simulink model "Model_3D"  (R2020b)
settings: Solver=ode8  StartTime=0.0  StopTime=3  FixedStep=0.005  RelTol=1e-3
values from neighbouring files (symbols this model uses):
  Am = [1 8 10]    [my_config_1213.mat]    (also in my_config_1219.mat)
  Bm = [1 10]    [my_config_1213.mat]    (also in my_config_1219.mat)
  cc = [1 0.92774349 0.86070798 0.79851622 0.74081822 0.68728928 0.63762815 0.59155536 0.54881164 0.50915642 0.47236655 0.43823499 ... (41 elements, 1x41)]    [my_config_1213.mat]    (also in my_config_1219.mat)
  cc_new = [1 0.92774349 0.86070798 0.79851622 0.74081822 0.68728928 0.63762815 0.59155536 0.54881164 0.50915642 0.47236655 0.43823499 ... (41 elements, 1x41)]    [my_config_1213.mat]    (also in my_config_1219.mat)
  D = [64.807 64.807 64.807]    [my_config_1213.mat]    (also in my_config_1219.mat)
  g1 = [-1 0 1]    [my_config_1213.mat]
  g2 = [-1 0.6 1]    [my_config_1213.mat]
  gamma1 = 1.2    [my_config_1213.mat]    (also in my_config_1219.mat)
  gamma2 = 0.5    [my_config_1213.mat]    (also in my_config_1219.mat)
  K = [1050 1050 1050]    [my_config_1213.mat]    (also in my_config_1219.mat; my_config_1224.mat)
  left_0 = [0 0 0]    [my_config_1219.mat]
  m1 = 1    [my_config_1213.mat]    (also in my_config_1219.mat; my_config_1224.mat)
  m2 = 1    [my_config_1213.mat]    (also in my_config_1219.mat; my_config_1224.mat)
  right_0 = [0 0.6 0]    [my_config_1213.mat]    (also in my_config_1219.mat)
  tau1 = 3    [my_config_1213.mat]    (also in my_config_1219.mat)
  weight = [0.0266866854 0.00199886353 0 0.185908993 0.0191898792 0 0.285018336 0.0372844837 0 0.420259935 0.0646488362 0 ... (123 elements, 3x41)]    [my_config_1213.mat]    (also in my_config_1219.mat)
  width = [191.53405062 222.53081866 258.54392519 300.38518553 348.99779456 405.47758835 471.09774681 547.33749391 635.91544276 738.82833688 858.39606128 997.31393782 ... (41 elements, 1x41)]    [my_config_1213.mat]    (also in my_config_1219.mat)
  width_new = [191.53405062 222.53081866 258.54392519 300.38518553 348.99779456 405.47758835 471.09774681 547.33749391 635.91544276 738.82833688 858.39606128 997.31393782 ... (41 elements, 1x41)]    [my_config_1213.mat]    (also in my_config_1219.mat)
  x1_0 = [0 0.2 0]    [my_config_1213.mat]    (also in my_config_1219.mat; my_config_1224.mat)
  x2_0 = [0 0.4 0]    [my_config_1213.mat]    (also in my_config_1219.mat; my_config_1224.mat)
undefined symbols (not defined in the file or in its folder): b1, b2, b3, k1, k2, k3
settings Model: Creator=nathan  LastModifiedBy=10788
settings OptimizationCC: DefaultParameterBehavior=Inlined  EnhancedBackFolding=on  PassReuseOutputArgsAs=Individual arguments  ZeroExternalMemoryAtStartup=off  ZeroInternalMemoryAtStartup=off  OptimizeBlockOrder=speed  DifferentSizesBufferReuse=on  OptimizationCustomize=off  EfficientTunableParamExpr=on
settings DebuggingCC: ParameterTunabilityLossMsg=error
settings SFSimCC: MATLABDynamicMemAlloc=off  SimTargetLang=C++
settings RTWCC: Description=Create Visual C/C++ Solution File for Embedded Coder  SystemTargetFile=ert.tlc  GenCodeOnly=on  TemplateMakefile=RTW.MSVCBuild  GenerateReport=on  IncludeHyperlinkInReport=on  LaunchReport=on  TargetLang=C++  GenerateTraceInfo=on  GenerateTraceReport=on  GenerateTraceReportSl=on  GenerateTraceReportSf=on  GenerateTraceReportEml=on
settings CodeAppCC: ForceParamTrailComments=on  IgnoreCustomStorageClasses=off  OperatorAnnotations=on  SimulinkDataObjDesc=on  SFDataObjDesc=on  InsertBlockDesc=on
settings ERTTargetCC: TargetLangStandard=C++03 (ISO)  GenerateSampleERTMain=on  CodeInterfacePackaging=C++ class  SupportContinuousTime=on  InlinedParameterPlacement=NonHierarchical  RootIOFormat=Structure reference  ERTCustomFileTemplate=example_file_process.tlc

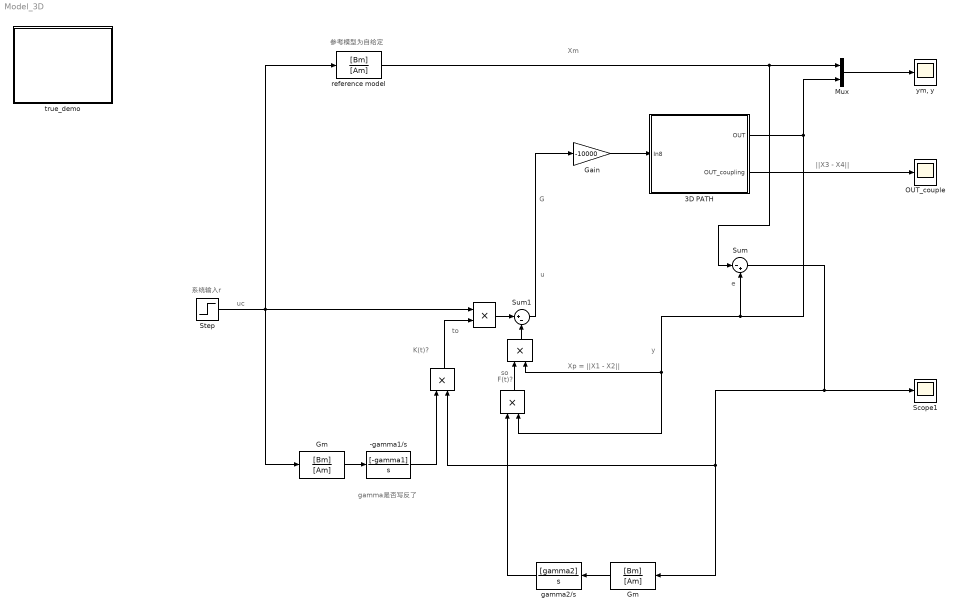
== system Model_3D ==
  note: 参考模型为自给定
  note: 系统输入r
  note: gamma是否写反了
  note: F(t)?
  note: K(t)?
  note: Xp = ||X1 - X2||
  note: ||X3 - X4||
  note: y
  note: u
  note: e
  note: so
  note: to
  note: uc
  note: Xm
  note: G
  " " : Product
  " " : Product
  "  " : Product
  "     " : Product
  -gamma1/s : TransferFcn  Numerator=[-gamma1]  Denominator=[1 0]
  3D PATH : Subsystem
  Gain : Gain  Gain=-10000
  "Gm " : TransferFcn  Numerator=[Bm]  Denominator=[Am]
  "Gm  " : TransferFcn  Numerator=[Bm]  Denominator=[Am]
  Mux : Mux  Inputs=2
  OUT_couple : Scope
  Scope1 : Scope
  Step : Step  Time=0  After=0.2  SampleTime=0
  Sum : Sum  Inputs=|-+
  Sum1 : Sum  Inputs=|+-
  gamma2/s : TransferFcn  Numerator=[gamma2]  Denominator=[1 0]
  reference model : TransferFcn  Numerator=[Bm]  Denominator=[Am]
  true_demo : Subsystem
  "ym, y" : Scope
  wires:
  3D PATH/1(OUT) -> "  "/2, " "/2, Sum/2, Mux/2
  " "/1 -> Sum1/2
  Step/1 -> "Gm  "/1, reference model/1, "     "/1
  "  "/1 -> " "/1
  Gain/1 -> 3D PATH/1(In8)
  Sum1/1 -> Gain/1
  -gamma1/s/1 -> " "/1
  " "/1 -> "     "/2
  "Gm "/1 -> gamma2/s/1
  "     "/1 -> Sum1/1
  reference model/1 -> Sum/1, Mux/1
  Mux/1 -> "ym, y"/1
  gamma2/s/1 -> "  "/1
  Sum/1 -> "Gm "/1, " "/2, Scope1/1
  "Gm  "/1 -> -gamma1/s/1
  3D PATH/2(OUT_coupling) -> OUT_couple/1

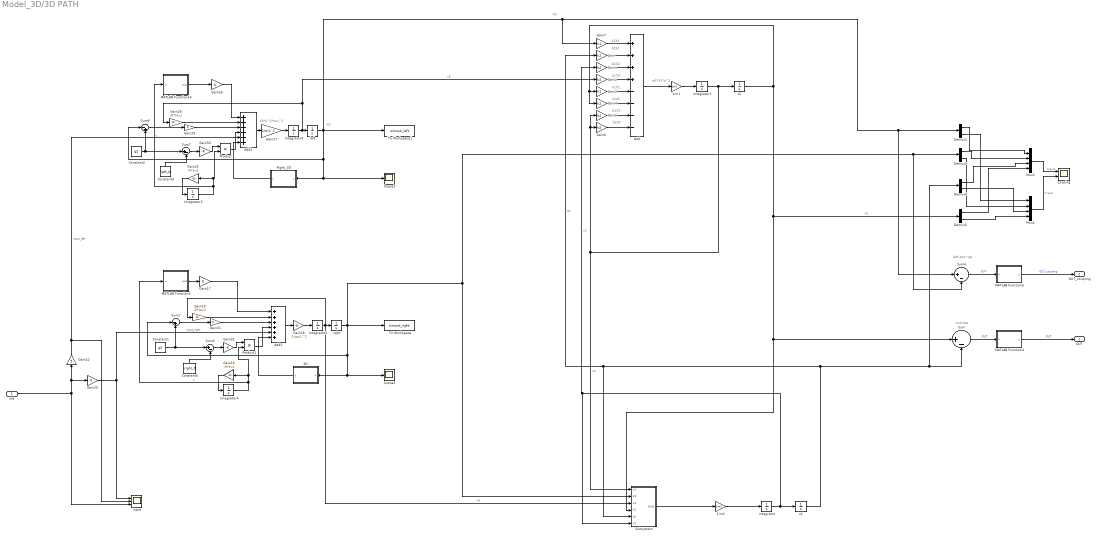
== system Model_3D/3D PATH ==
  note: X3*s^2*tau^2
  note: m1*X1*s^2
  note: k1X3
  note: X3
  note: mid two
  note: left and rigt
  note: X3
  note: k2X2
  note: b2X2'
  note: b1X3'
  note: k1X1
  note: k2X1
  note: b1X1'
  note: b2X1'
  In8 : Inport
  1/m1 : Gain  Gain=1/m1
  1/m2 : Gain  Gain=1/m2
  3D : MATLAB Function  TreatAsAtomicUnit=on
  Add : Sum  Inputs=++++----
  Add2 : Sum  Inputs=++++++
  Add4 : Sum  Inputs=++++++
  Constant1 : Constant  Value=g2
  Constant2 : Constant  Value=g1
  Constant4 : Constant  Value=left_0
  Constant5 : Constant  Value=right_0
  Demux{2..5} (4 alike) : Demux  Outputs=2
  Gain : Gain  Gain=k2
  Gain1 : Gain  Gain=b2
  Gain16 : Gain  Gain=-3/tau1
  Gain{17,26,29,31} (4 alike) : Gain  Gain=K
  Gain18 : Gain  Gain=1/tau1^2
  Gain19 : Gain  Gain=-D*tau1
  Gain2 : Gain  Gain=b1
  Gain20 : Gain  Gain=-5
  Gain22 : Gain  Gain=5
  Gain25 : Gain  Gain=-3/tau1
  Gain27 : Gain  Gain=1/tau1^2
  Gain28 : Gain  Gain=-D*tau1
  Gain3 : Gain  Gain=k1
  Gain30 : Gain  Gain=-K
  Gain32 : Gain  Gain=-K
  Gain4 : Gain  Gain=k2
  Gain5 : Gain  Gain=b1
  Gain6 : Gain  Gain=b2
  Gain7 : Gain  Gain=k1
  Integrator{,1,3,5} (4 alike) : Integrator
  Integrator2 : Integrator  InitialCondition=1
  Integrator4 : Integrator  InitialCondition=1
  MATLAB Function14 : MATLAB Function  TreatAsAtomicUnit=on
  MATLAB Function2 : MATLAB Function  TreatAsAtomicUnit=on
  MATLAB Function4 : MATLAB Function  TreatAsAtomicUnit=on
  MATLAB Function5 : MATLAB Function  TreatAsAtomicUnit=on
  Mux3 : Mux
  Mux4 : Mux
  Product : Product
  Product1 : Product
  Right_3D : MATLAB Function  TreatAsAtomicUnit=on
  Scope3 : Scope
  Scope4 : Scope
  Subsystem : Subsystem
  Sum{,3..4,7} (4 alike) : Sum  Inputs=|+-
  Sum2 : Sum  Inputs=|-+
  Sum6 : Sum  Inputs=|-+
  To Workspace : ToWorkspace  VariableName=simout_right  SaveFormat=Timeseries  SampleTime=-1
  To Workspace1 : ToWorkspace  VariableName=simout_left  SaveFormat=Timeseries  SampleTime=-1
  couping : Scope  NumInputPorts=2
  input : Scope  NumInputPorts=3
  left : Integrator  InitialCondition=left_0
  right : Integrator  InitialCondition=right_0
  x1 : Integrator  InitialCondition=x1_0
  x2 : Integrator  InitialCondition=x2_0
  OUT : Outport
  OUT_coupling : Outport  Port=2
  wires:
  Add/1 -> 1/m1/1
  Gain22/1 -> Add4/5, input/2  "input_left"
  Gain/1 -> Add/2
  Integrator5/1 -> Subsystem/3(x4'), right/1, Gain19/1  "x4'"
  Demux2/1 -> Mux3/1
  x2/1 -> Demux4/1, Sum/2, Subsystem/5(X2), Gain/1  "X2"
  Integrator/1 -> x2/1, Subsystem/6(x2'), Gain1/1  "x2'"
  Gain20/1 -> input/1, Add2/5  "input_right"
  MATLAB Function5/1(y) -> OUT_coupling/1  "OUT_coupling"
  left/1 -> Right_3D/1(u), Scope3/1, Sum6/1, To Workspace1/1, Sum4/1, Demux2/1, Gain7/1
  MATLAB Function14/1(out) -> Gain26/1
  MATLAB Function2/1(out) -> Gain17/1
  Gain7/1 -> Add/1
  Add2/1 -> Gain18/1
  1/m2/1 -> Integrator/1
  Gain5/1 -> Add/7
  Gain19/1 -> Add2/2
  Constant1/1 -> Sum3/1, Sum2/2
  Integrator1/1 -> x1/1, Subsystem/1(x1'), Gain5/1, Gain6/1  "x1'"
  Gain30/1 -> Product/1
  Constant2/1 -> Sum7/1, Sum6/2
  Sum6/1 -> Gain29/1
  Mux3/1 -> couping/1  "X axis"
  Gain32/1 -> Product1/1
  Gain3/1 -> Add/5
  In8/1 -> input/3, Gain22/1, Gain20/1
  Mux4/1 -> couping/2  "Y axis"
  Demux5/2 -> Mux4/4
  Sum7/1 -> Gain30/1
  Integrator2/1 -> MATLAB Function14/1(u), Product/2, Gain25/1  "s"
  right/1 -> Scope4/1, 3D/1(u), Sum2/1, To Workspace/1, Subsystem/2(In2), Sum4/2, Demux3/1
  Gain16/1 -> Integrator4/1
  Gain28/1 -> Add4/2
  Demux5/1 -> Mux3/4
  Demux4/1 -> Mux3/3
  Gain2/1 -> Add/4
  Product/1 -> Add4/4
  Gain29/1 -> Add4/3
  Gain27/1 -> Integrator3/1
  Integrator3/1 -> Gain2/1, Gain28/1, left/1  "x3'"
  x1/1 -> Gain4/1, Gain3/1, Subsystem/4(X1), Sum/1, Demux5/1  "X1"
  Demux3/1 -> Mux3/2
  Gain1/1 -> Add/3
  Integrator4/1 -> Product1/2, Gain16/1, MATLAB Function2/1(u)  "s"
  Gain17/1 -> Add2/1
  Gain26/1 -> Add4/1
  Sum4/1 -> MATLAB Function5/1(u)  "OUT"
  Demux4/2 -> Mux4/3
  Constant5/1 -> Sum3/2
  Gain18/1 -> Integrator5/1
  Demux3/2 -> Mux4/2
  3D/1(y) -> Add2/6
  Demux2/2 -> Mux4/1
  Product1/1 -> Add2/4
  Gain6/1 -> Add/8
  Gain31/1 -> Add2/3
  Sum2/1 -> Gain31/1
  1/m1/1 -> Integrator1/1
  Gain4/1 -> Add/6
  Gain25/1 -> Integrator2/1
  Sum/1 -> MATLAB Function4/1(u)  "OUT"
  Sum3/1 -> Gain32/1
  Add4/1 -> Gain27/1
  Constant4/1 -> Sum7/2
  Right_3D/1(y) -> Add4/6
  MATLAB Function4/1(y) -> OUT/1  "OUT"
  Subsystem/1(Out1) -> 1/m2/1

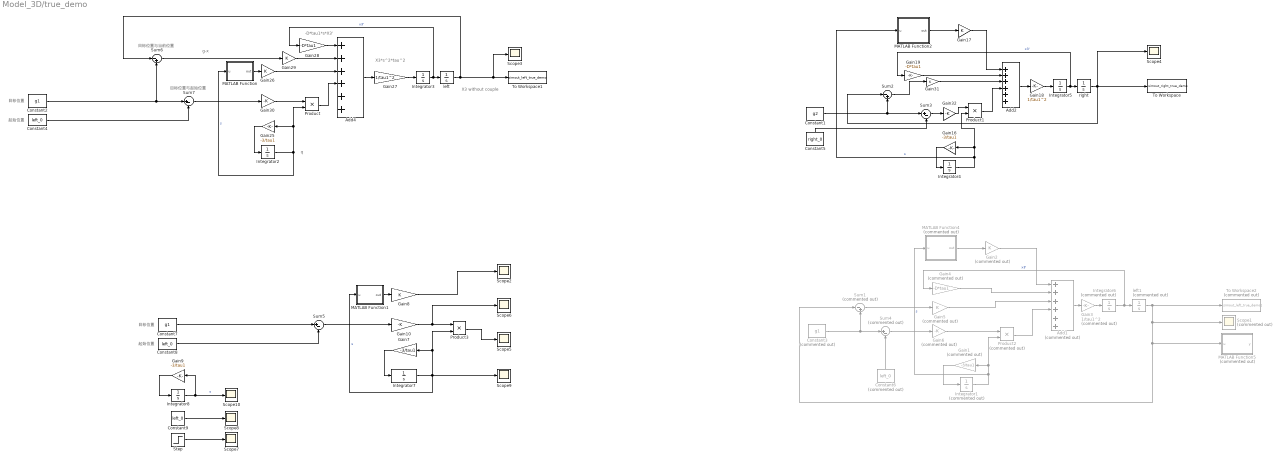
== system Model_3D/true_demo ==
  note: -D*tau1*s*X3'
  note: X3*s^2*tau^2
  note: g-x
  note: X3 without couple
  note: 目标位置与起始位置
  note: 目标位置
  note: 起始位置
  note: 目标位置与当前位置
  note: 目标位置
  note: 起始位置
  note: q
  Add1 : Sum  Commented=on  Inputs=++++++
  Add2 : Sum  Inputs=++++++
  Add4 : Sum  Inputs=++++++
  Constant1 : Constant  Value=g2
  Constant2 : Constant  Value=g1
  Constant3 : Constant  Commented=on  Value=g1
  Constant4 : Constant  Value=left_0
  Constant5 : Constant  Value=right_0
  Constant6 : Constant  Commented=on  Value=left_0
  Constant7 : Constant  Value=g1
  Constant8 : Constant  Value=left_0
  Constant9 : Constant  Value=left_0
  Gain1 : Gain  Commented=on  Gain=-3/tau1
  Gain10 : Gain  Gain=-K
  Gain{7,9,16,25} (4 alike) : Gain  Gain=-3/tau1
  Gain{8,17,26,29,31} (5 alike) : Gain  Gain=K
  Gain18 : Gain  Gain=1/tau1^2
  Gain19 : Gain  Gain=-D*tau1
  Gain2 : Gain  Commented=on  Gain=K
  Gain27 : Gain  Gain=1/tau1^2
  Gain28 : Gain  Gain=-D*tau1
  Gain3 : Gain  Commented=on  Gain=1/tau1^2
  Gain30 : Gain  Gain=-K
  Gain32 : Gain  Gain=-K
  Gain4 : Gain  Commented=on  Gain=-D*tau1
  Gain5 : Gain  Commented=on  Gain=K
  Gain6 : Gain  Commented=on  Gain=-K
  Integrator1 : Integrator  Commented=on  InitialCondition=1
  Integrator{2,4,7..8} (4 alike) : Integrator  InitialCondition=1
  Integrator3 : Integrator
  Integrator5 : Integrator
  Integrator6 : Integrator  Commented=on
  MATLAB Function : MATLAB Function  TreatAsAtomicUnit=on
  MATLAB Function1 : MATLAB Function  TreatAsAtomicUnit=on
  MATLAB Function2 : MATLAB Function  TreatAsAtomicUnit=on
  MATLAB Function4 : MATLAB Function  Commented=on  TreatAsAtomicUnit=on
  MATLAB Function5 : MATLAB Function  Commented=on  TreatAsAtomicUnit=on
  Product : Product
  Product1 : Product
  Product2 : Product  Commented=on
  Product3 : Product
  Scope1 : Scope  Commented=on
  Scope{2..10} (9 alike) : Scope
  Step : Step  Time=0  After=0.2  SampleTime=0
  Sum1 : Sum  Commented=on  Inputs=|-+
  Sum2 : Sum  Inputs=|-+
  Sum3 : Sum  Inputs=|+-
  Sum4 : Sum  Commented=on  Inputs=|+-
  Sum5 : Sum  Inputs=|+-
  Sum6 : Sum  Inputs=|-+
  Sum7 : Sum  Inputs=|+-
  To Workspace : ToWorkspace  VariableName=simout_right_true_demo  SaveFormat=Timeseries  SampleTime=-1
  To Workspace1 : ToWorkspace  VariableName=simout_left_true_demo  SaveFormat=Timeseries  SampleTime=-1
  To Workspace2 : ToWorkspace  Commented=on  VariableName=simout_left_true_demo1  SaveFormat=Timeseries  SampleTime=-1
  left : Integrator  InitialCondition=left_0
  left1 : Integrator  Commented=on  InitialCondition=left_0
  right : Integrator  InitialCondition=right_0
  wires:
  Integrator5/1 -> right/1, Gain19/1  "x3'"
  left/1 -> Sum6/1, Scope3/1, To Workspace1/1
  MATLAB Function/1(out) -> Gain26/1
  MATLAB Function2/1(out) -> Gain17/1
  Add2/1 -> Gain18/1
  Gain19/1 -> Add2/2
  Constant1/1 -> Sum2/2, Sum3/1
  Gain30/1 -> Product/1
  Constant2/1 -> Sum7/1, Sum6/2
  Sum6/1 -> Gain29/1
  Gain32/1 -> Product1/1
  Sum7/1 -> Gain30/1
  Integrator2/1 -> Product/2, Gain25/1, MATLAB Function/1(u)  "s"
  right/1 -> Sum2/1, Scope4/1, To Workspace/1
  Gain16/1 -> Integrator4/1
  Product/1 -> Add4/4
  Gain27/1 -> Integrator3/1
  Integrator3/1 -> Gain28/1, left/1  "x3'"
  Integrator4/1 -> Product1/2, Gain16/1, MATLAB Function2/1(u)  "s"
  Gain17/1 -> Add2/1
  Constant5/1 -> Sum3/2
  Gain18/1 -> Integrator5/1
  Product1/1 -> Add2/4
  Gain31/1 -> Add2/3
  Sum2/1 -> Gain31/1
  Gain25/1 -> Integrator2/1
  Sum3/1 -> Gain32/1
  Add4/1 -> Gain27/1
  Constant4/1 -> Sum7/2
  Add1/1 -> Gain3/1
  left1/1 -> To Workspace2/1, Scope1/1, MATLAB Function5/1(u), Sum1/1
  Gain2/1 -> Add1/1
  Gain6/1 -> Product2/1
  Constant6/1 -> Sum4/2
  Gain4/1 -> Add1/2
  Integrator6/1 -> Gain4/1, left1/1  "x3'"
  Integrator1/1 -> MATLAB Function4/1(u), Product2/2, Gain1/1  "s"
  Sum4/1 -> Gain6/1
  Gain5/1 -> Add1/3
  Constant3/1 -> Sum1/2, Sum4/1
  Sum1/1 -> Gain5/1
  Gain1/1 -> Integrator1/1
  Gain3/1 -> Integrator6/1
  MATLAB Function4/1(out) -> Gain2/1
  Product2/1 -> Add1/4
  Gain28/1 -> Add4/1
  Gain29/1 -> Add4/2
  Gain26/1 -> Add4/3
  Gain8/1 -> Scope2/1
  Product3/1 -> Scope5/1
  Gain7/1 -> Integrator7/1
  Constant7/1 -> Sum5/1
  Integrator7/1 -> MATLAB Function1/1(u), Scope9/1, Product3/2, Gain7/1  "s"
  MATLAB Function1/1(out) -> Gain8/1
  Constant8/1 -> Sum5/2
  Sum5/1 -> Gain10/1
  Gain10/1 -> Scope6/1, Product3/1
  Step/1 -> Scope7/1
  Constant9/1 -> Scope8/1
  Integrator8/1 -> Gain9/1, Scope10/1  "s"
  Gain9/1 -> Integrator8/1

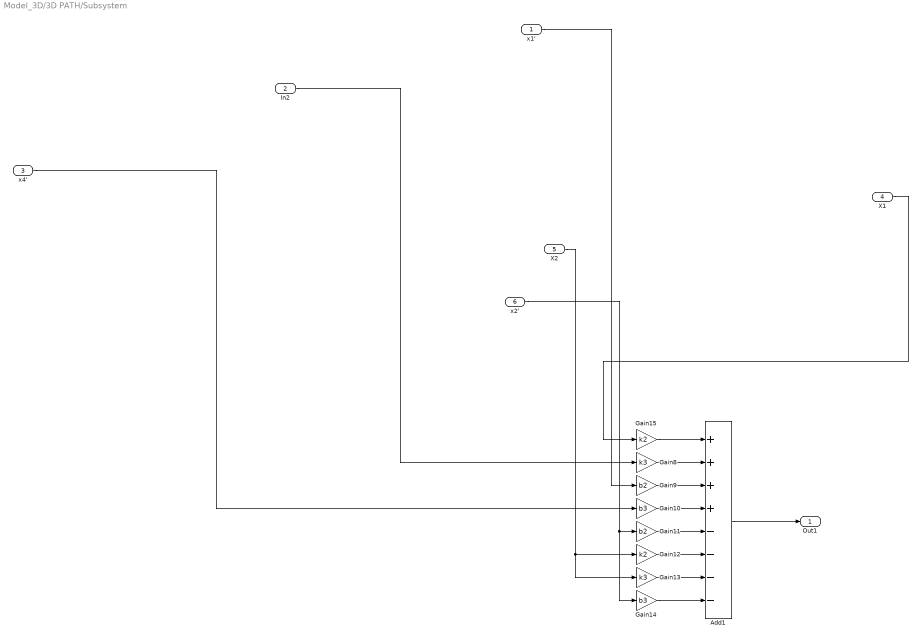
== system Model_3D/3D PATH/Subsystem ==
  x1' : Inport
  In2 : Inport  Port=2
  x4' : Inport  Port=3
  X1 : Inport  Port=4
  X2 : Inport  Port=5
  x2' : Inport  Port=6
  Add1 : Sum  Inputs=++++----
  Gain10 : Gain  Gain=b3
  Gain11 : Gain  Gain=b2
  Gain12 : Gain  Gain=k2
  Gain13 : Gain  Gain=k3
  Gain14 : Gain  Gain=b3
  Gain15 : Gain  Gain=k2
  Gain8 : Gain  Gain=k3
  Gain9 : Gain  Gain=b2
  Out1 : Outport
  wires:
  Gain8/1 -> Add1/2
  Gain10/1 -> Add1/4
  x2'/1 -> Gain14/1, Gain11/1
  Gain13/1 -> Add1/7
  X1/1 -> Gain15/1
  Gain12/1 -> Add1/6
  X2/1 -> Gain12/1, Gain13/1
  Gain9/1 -> Add1/3
  Gain14/1 -> Add1/8
  Gain15/1 -> Add1/1
  Gain11/1 -> Add1/5
  x1'/1 -> Gain9/1
  x4'/1 -> Gain10/1
  In2/1 -> Gain8/1
  Add1/1 -> Out1/1

== matlab function Model_3D/3D PATH/Right_3D ==
  data: u input; y output
function y = fcn(u)

n_dim=3;
n_obt=1;
phi=zeros(n_dim,1);
phi_tal=zeros(n_dim,1);

x_c_1 = 0.15;
y_c_1 = 0.2;
z_c_1 = 0.4;
a_1 = .1;
b_1 = .1;
c_1 = .1;

x_c_2 = -0.4;
y_c_2 = 1.1;
z_c_2 = 0.8;
a_2 = 0.15;
b_2 = 0.15;
c_2 = .2;

% center=[x_c_1 y_c_1;
%     x_c_2 y_c_2];
% axis=[a_1 b_1;
%     a_2 b_2];

center=[x_c_1 y_c_1 z_c_1;
    x_c_2 y_c_2 z_c_2
];
axis=[a_1 b_1 c_1;
    a_2 b_2 c_2
];

% center=center(:,[2 1]);
% axis=axis(:,[2 1]);

%%%%%%%%%%%%%

for j=1:n_obt
    
    
    K = 0;
for i = 1:n_dim
    
    K =K+( (u(i) - center(j,i)) / axis(j,i)) ^2;
    
end
K = K - 1;

for i = 1:n_dim
    phi(i) = (u(i) - center(j,i)) / axis(j,i) ^2;
   
end

phi =phi * ( exp(-K)) * (1 / K + 1 / K / K) * 2;
      
phi_tal=phi_tal+phi;
end


y = phi_tal;

== matlab function Model_3D/true_demo/MATLAB Function4 ==
  data: u input; out output; width_new parameter; weight parameter; cc_new parameter
function out = fcn(u, width_new, weight, cc_new)


% if(u>2.5)
%     y=1;
% elseif(u>=0&&u<=2.5)
%     y=0;
% else
%         y=-1;
% end


tem=exp(-width_new.*(u-cc_new).^2)';
y=(weight*tem*u)/sum(tem) ;

out = y;

== matlab function Model_3D/true_demo/MATLAB Function5 ==
  data: u input; y output
function y = fcn(u)

n_dim=2;
n_obt=1;
phi=zeros(n_dim,1);
phi_tal=zeros(n_dim,1);
x_c_1 = -0.7;
y_c_1 = 0.4;
a_1 = .2;
b_1 = .2;

x_c_2 = 0.15;
y_c_2 = 0.4;
a_2 = 0.1;
b_2 = 0.1;


center=[x_c_1 y_c_1;
    x_c_2 y_c_2];
axis=[a_1 b_1;
    a_2 b_2];

% center=center(:,[2 1]);
% axis=axis(:,[2 1]);

%%%%%%%%%%%%%

for j=1:n_obt
    
    
    K = 0;
for i = 1:n_dim
    
    K =K+( (u(i) - center(j,i)) / axis(j,i)) ^2;
    
end
K = K - 1;

for i = 1:n_dim
    phi(i) = (u(i) - center(j,i)) / axis(j,i) ^2;
   
end

phi =phi * ( exp(-K)) * (1 / K + 1 / K / K) * 2;
      
phi_tal=phi_tal+phi;
end


y = phi_tal;

== matlab function Model_3D/true_demo/MATLAB Function1 ==
  data: u input; out output; width_new parameter; weight parameter; cc_new parameter
function out = fcn(u, width_new, weight, cc_new)

% if(u>2.5)
%     y=1;
% elseif(u>=0&&u<=2.5)
%     y=0;
% else
%         y=-1;
% end

tem=exp(-width_new.*(u-cc_new).^2)';
y=(weight*tem*u)/sum(tem) ;

out = y;

== matlab function Model_3D/true_demo/MATLAB Function ==
  data: u input; out output; width_new parameter; weight parameter; cc_new parameter
function out = fcn(u, width_new, weight, cc_new)


% if(u>2.5)
%     y=1;
% elseif(u>=0&&u<=2.5)
%     y=0;
% else
%         y=-1;
% end


tem=exp(-width_new.*(u-cc_new).^2)';
y=(weight * tem * u) / sum(tem) ;

out = y;

== matlab function Model_3D/true_demo/MATLAB Function2 ==
  data: u input; out output; width parameter; weight parameter; cc parameter
function out = fcn(u, width, weight, cc)


% if(u>2.5)
%     y=1;
% elseif(u>=0&&u<=2.5)
%     y=0;
% else
%         y=-1;
% end


tem=exp(-width.*(u-cc).^2)';
y=(weight*tem*u)/sum(tem) ;

out = y;

== matlab function Model_3D/3D PATH/3D ==
  data: u input; y output
function y = fcn(u)

n_dim=3;
n_obt=2;
phi=zeros(n_dim,1);     % 3行1列
phi_tal=zeros(n_dim,1); % 2行1列

% 障碍物1
x_c_1 = 0.2;
y_c_1 = 0.8;
z_c_1 = 0.4;
a_1 = .1;
b_1 = .2;
c_1 = .1;

% 障碍物2
x_c_2 = -0.4;
y_c_2 = 1.2;
z_c_2 = 0.8;
a_2 = 0.15;
b_2 = 0.15;
c_2 = .2;

center=[x_c_1 y_c_1 z_c_1;
    x_c_2 y_c_2 z_c_2
];
axis=[a_1 b_1 c_1;
    a_2 b_2 c_2
];

% center=center(:,[2 1]);
% axis=axis(:,[2 1]);

%%%%%%%%%%%%%

for j=1:n_obt % 障碍物数量
    K = 0;
    for i = 1:n_dim % 坐标维度
        K =K+( (u(i) - center(j,i)) / axis(j,i)) ^2;
    end
    K = K - 1;

    for i = 1:n_dim
        phi(i) = (u(i) - center(j,i)) / axis(j,i) ^2;
    end

    phi = phi * ( exp(-K)) * (1 / K + 1 / K / K) * 2;
    phi_tal=phi_tal+phi;
end

y = phi_tal;

== matlab function Model_3D/3D PATH/MATLAB Function14 ==
  data: u input; out output; width parameter; weight parameter; cc parameter
function out = fcn(u, width, weight, cc)


% if(u>2.5)
%     y=1;
% elseif(u>=0&&u<=2.5)
%     y=0;
% else
%         y=-1;
% end


tem=exp(-width.*(u-cc).^2)';
y=(weight*tem*u)/sum(tem) ;

out = y;

== matlab function Model_3D/3D PATH/MATLAB Function2 ==
  data: u input; out output; width parameter; weight parameter; cc parameter
function out = fcn(u, width, weight, cc)


% if(u>2.5)
%     y=1;
% elseif(u>=0&&u<=2.5)
%     y=0;
% else
%         y=-1;
% end


tem=exp(-width.*(u-cc).^2)';
y=(weight*tem*u)/sum(tem) ;

out = y;

== matlab function Model_3D/3D PATH/MATLAB Function4 ==
  data: u input; y output
function y = fcn(u)

y = norm(u);

== matlab function Model_3D/3D PATH/MATLAB Function5 ==
  data: u input; y output
function y = fcn(u)

y = norm(u);
